simulink model "x20240109_HVDCMMCInterconnection"  (R2023b)
settings: Solver=FixedStepDiscrete  StartTime=0.0  StopTime=2  FixedStep=Ts_Power  RelTol=1e-4  EnableMultiTasking=on
PreLoadFcn:
  | HVDCMMCInterconnectionParam
StartFcn:
  | tic
StopFcn:
  | toc
values from neighbouring files (symbols this model uses):
  C_PM = 1.758e-3    (= 0.001758)    [HVDCMMCInterconnectionParam.m]
  Cg = 50e-9    (= 5e-08)    [HVDCMMCInterconnectionParam.m]
  D_R = 0.001    [HVDCMMCInterconnectionParam.m]
  D_Rs = 1e8    (= 100000000)    [HVDCMMCInterconnectionParam.m]
  D_Vf = 0    [HVDCMMCInterconnectionParam.m]
  Fnom = 50    [HVDCMMCInterconnectionParam.m]
  HRM = 2    [HVDCMMCInterconnectionParam.m]
  Ki_Ireg = 6    [HVDCMMCInterconnectionParam.m]
  Ki_Preg = 1.0    (= 1)    [HVDCMMCInterconnectionParam.m]
  Ki_Qreg = 1.0    (= 1)    [HVDCMMCInterconnectionParam.m]
  Ki_VDCreg = 100    [HVDCMMCInterconnectionParam.m]
  Kp_Ireg = 0.6    [HVDCMMCInterconnectionParam.m]
  Kp_Preg = 0.5/3    (= 0.166666666667)    [HVDCMMCInterconnectionParam.m]
  Kp_Qreg = 0.5/3    (= 0.166666666667)    [HVDCMMCInterconnectionParam.m]
  Kp_VDCreg = 4    [HVDCMMCInterconnectionParam.m]
  L_cable = 15e-3    (= 0.015)    [HVDCMMCInterconnectionParam.m]
  Larm = Larm_pu*(Zb_ac/(2*pi*Fnom))    [HVDCMMCInterconnectionParam.m]
  Lff = Larm_pu/2    (= 0.075)    [HVDCMMCInterconnectionParam.m]
  Limits_Ireg = [ 2.0  -2.0]    [HVDCMMCInterconnectionParam.m]
  Limits_Preg = [ 1.2, 0.8 ]    [HVDCMMCInterconnectionParam.m]
  Limits_Qreg = [ 0.25, -0.25 ]    [HVDCMMCInterconnectionParam.m]
  Limits_VDCreg = [ 2.0  -2.0]    [HVDCMMCInterconnectionParam.m]
  Lxfo = 0.12    [HVDCMMCInterconnectionParam.m]
  Nb_PM = 36    [HVDCMMCInterconnectionParam.m]
  Pnom = 1000e6    (= 1000000000)    [HVDCMMCInterconnectionParam.m]
  R_cable = 0.5    [HVDCMMCInterconnectionParam.m]
  R_startup = 400    [HVDCMMCInterconnectionParam.m]
  Rarm = Rarm_pu*Zb_ac    [HVDCMMCInterconnectionParam.m]
  Rff = Rarm_pu/2    (= 0.00075)    [HVDCMMCInterconnectionParam.m]
  Rg = 100    [HVDCMMCInterconnectionParam.m]
  Rxfo = 0.003    [HVDCMMCInterconnectionParam.m]
  Slope_Pref = 0.5    [HVDCMMCInterconnectionParam.m]
  Slope_Qref = 0.5    [HVDCMMCInterconnectionParam.m]
  Slope_Vdc_ref = Vnom_dc/5    (= 128000)    [HVDCMMCInterconnectionParam.m]
  Tbrk1_On = 0.1    [HVDCMMCInterconnectionParam.m]
  Tbrk2_On = 1.0    (= 1)    [HVDCMMCInterconnectionParam.m]
  Tdeblock = 1.5    [HVDCMMCInterconnectionParam.m]
  Tfault = 9999    [HVDCMMCInterconnectionParam.m]
  Ton_Converter2 = 4    [HVDCMMCInterconnectionParam.m]
  Ton_PQreg = 4    [HVDCMMCInterconnectionParam.m]
  Ton_VDCreg = 1.5    [HVDCMMCInterconnectionParam.m]
  Ts = Ts_Control    (= 4e-05)    [HVDCMMCInterconnectionParam.m]
  Ts_Control = 40e-6    (= 4e-05)    [HVDCMMCInterconnectionParam.m]
  Ts_Power = 20e-6    (= 2e-05)    [HVDCMMCInterconnectionParam.m]
  Vb_ac = sqrt(2/3)*Vnom_sec    [HVDCMMCInterconnectionParam.m]
  Vb_dc = Vnom_dc    (= 640000)    [HVDCMMCInterconnectionParam.m]
  Vc0_PM = 0    [HVDCMMCInterconnectionParam.m]
  Vnom_dc = 640e3    (= 640000)    [HVDCMMCInterconnectionParam.m]
  Vnom_prim = 400e3    (= 400000)    [HVDCMMCInterconnectionParam.m]
  Vnom_sec = 333e3    (= 333000)    [HVDCMMCInterconnectionParam.m]
  w = 2*pi*Fnom    (= 314.159265359)    [HVDCMMCInterconnectionParam.m]
undefined symbols (not defined in the file or in its folder): DiscIntNeverNeededParam, gcbh, Pcc, S, sps_AC, sps_ACDC2, sps_rtmsupport
libraries: simulink x48, spsControlledVoltageSourceLib x30, spsCurrentMeasurementLib x30, MMC_Lib x30, spsDiodeLib x20, spsSeriesRLCBranchLib x14, powerlib_extras x12, spsVoltageMeasurementLib x12, spsSecondOrderFilterLib x8, spsabctodq0Lib x8, spsGroundLib x7, spsMeanLib x4
(part 7 of 9)

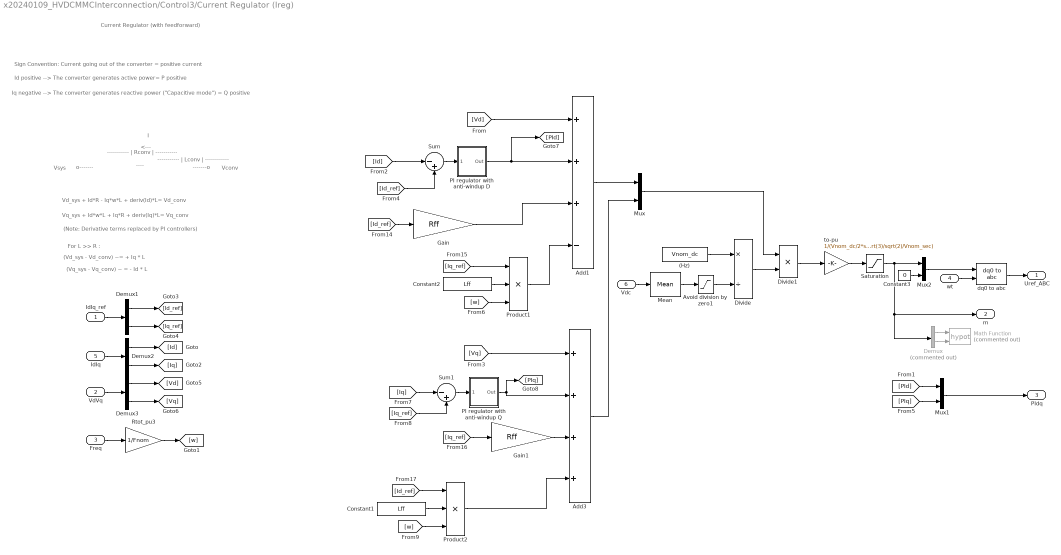
== system x20240109_HVDCMMCInterconnection/Control3/Current Regulator (Ireg) ==
  note: -----------
      | | Lconv |
      | ------------
  note: <---
  note: -------o
  note: Vconv
  note: ----
  note: -----------
      | | Rconv |
      | -----------
  note: For L >> R :
  note: (Vq_sys - Vq_conv) ~ = - Id * L
  note: (Vd_sys - Vd_conv) ~= + Iq * L
  note: Id positive --> The converter generates active power= P positive
  note: Iq negative --> The converter generates reactive power ("Capacitive mode") = Q positive
  note: Sign Convention: Current going out of the converter = positive current
  note: Current Regulator
      | (with feedforward)
  note: Vq_sys + Id*w*L + Iq*R + deriv(Iq)*L= Vq_conv
  note: Vd_sys + Id*R - Iq*w*L + deriv(Id)*L= Vd_conv
  note: (Note: Derivative terms replaced by PI controllers)
  note: Vsys
  note: o-------
  note: I
  IdIq_ref : Inport  PortDimensions=2
  VdVq : Inport  Port=2  PortDimensions=2
  Freq : Inport  Port=3  PortDimensions=1
  wt : Inport  Port=4  PortDimensions=1
  IdIq : Inport  Port=5  PortDimensions=2
  Vdc : Inport  Port=6  PortDimensions=1
  " (Hz)" : Constant  Value=Vnom_dc  SampleTime=Ts
  Add1 : Sum  Inputs=+++-
  Add3 : Sum  Inputs=++++
  Avoid division by zero1 : Saturate  UpperLimit=Vnom_dc*1.25  LowerLimit=Vnom_dc*0.75
  Constant1 : Constant  Value=Lff  SampleTime=Ts_Control
  Constant2 : Constant  Value=Lff  SampleTime=Ts_Control
  Constant3 : Constant  Value=0  SampleTime=Ts
  Demux : Demux  Commented=on  Outputs=2
  Demux1 : Demux  Outputs=2
  Demux2 : Demux  Outputs=2
  Demux3 : Demux  Outputs=2
  Divide : Product  Inputs=*/
  Divide1 : Product  Inputs=**
  Gain : Gain  Gain=Rff
  Gain1 : Gain  Gain=Rff
  Math Function : Math  Commented=on  Operator=hypot  SignedPower=on
  Mean : spsMeanLib/Mean  Freq=Fnom/3  Vinit=Vnom_dc  Ts=Ts
  Mux : Mux  Inputs=2
  Mux1 : Mux  Inputs=2
  Mux2 : Mux  Inputs=[2 1]
  PI regulator with anti-windup D : Subsystem  DialogController=POWERSYS.PowerSysDialog  mask(Discrete PI Controller){Kp=Kp_Ireg, Ki=Ki_Ireg, Par_Limits=Limits_Ireg, Init=0, Ts=Ts}
      mask prompts: Kp "Proportional gain (Kp):"; Ki "Integral gain (Ki):"; Par_Limits "Output limits: [ Upper   Lower ]"; Init "Output initial value:"; Ts "Sample time:"
      mask help: This block implements a discrete PI controller.
      mask init:
      | UpperLimit=Par_Limits(1);
      | LowerLimit=Par_Limits(2);
      | power_initmask();
      mask Help: This block is part of a subset of blocks in the Extras library that does not have documentation associated with it, other than the block mask description.
      mask Display: disp('PI');
  PI regulator with anti-windup Q : Subsystem  DialogController=POWERSYS.PowerSysDialog  mask(Discrete PI Controller){Kp=Kp_Ireg, Ki=Ki_Ireg, Par_Limits=Limits_Ireg, Init=0, Ts=Ts}
      mask prompts: Kp "Proportional gain (Kp):"; Ki "Integral gain (Ki):"; Par_Limits "Output limits: [ Upper   Lower ]"; Init "Output initial value:"; Ts "Sample time:"
      mask help: This block implements a discrete PI controller.
      mask init:
      | UpperLimit=Par_Limits(1);
      | LowerLimit=Par_Limits(2);
      | power_initmask();
      mask Help: This block is part of a subset of blocks in the Extras library that does not have documentation associated with it, other than the block mask description.
      mask Display: disp('PI');
  Product1 : Product  Inputs=3  RndMeth=Zero
  Product2 : Product  Inputs=3  RndMeth=Zero
  Rtot_pu3 : Gain  Gain=1/Fnom  SaturateOnIntegerOverflow=on  OutDataTypeStr=Inherit: Same as input  ParamDataTypeStr=Inherit: Same as input
  Saturation : Saturate  UpperLimit=Limits_Ireg(1)  LowerLimit=Limits_Ireg(2)
  Sum : Sum  Inputs=|-+
  Sum1 : Sum  Inputs=|-+
  dq0 to abc : spsdq0toabcLib/dq0 to abc  Alignment=90 degrees behind phase A axis
  to-pu : Gain  Gain=1/(Vnom_dc/2*sqrt(3)/sqrt(2)/Vnom_sec)
  Uref_ABC : Outport
  m : Outport  Port=2
  PIdq : Outport  Port=3
  wires:
  wt/1 -> dq0 to abc/2
  to-pu/1 -> Saturation/1
  Mux/1 -> Divide1/1
  dq0 to abc/1 -> Uref_ABC/1
  Divide/1 -> Divide1/2
  Mean/1 -> Avoid division by zero1/1
  Divide1/1 -> to-pu/1
  " (Hz)"/1 -> Divide/1
  Vdc/1 -> Mean/1
  Avoid division by zero1/1 -> Divide/2
  Mux1/1 -> PIdq/1
  Constant3/1 -> Mux2/2
  Mux2/1 -> dq0 to abc/1
  Demux/2 -> Math Function/2
  Demux/1 -> Math Function/1
  Saturation/1 -> Mux2/1, m/1, Demux/1
  PI regulator with anti-windup D/1(Out) -> [PId], Add1/2
  PI regulator with anti-windup Q/1(Out) -> [PIq], Add3/2
  [Vd] -> Add1/1
  Product1/1 -> Add1/4
  Gain/1 -> Add1/3
  Gain1/1 -> Add3/3
  Product2/1 -> Add3/4
  [Vq] -> Add3/1
  Demux2/1 -> [Id]
  IdIq/1 -> Demux2/1
  [Id_ref] -> Product2/1
  [Iq_ref] -> Gain1/1
  [Iq_ref] -> Product1/1
  [Id_ref] -> Gain/1
  [Id] -> Sum/1
  [Iq] -> Sum1/1
  Demux2/2 -> [Iq]
  [PIq] -> Mux1/2
  [PId] -> Mux1/1
  [w] -> Product1/3
  Constant2/1 -> Product1/2
  [w] -> Product2/3
  Constant1/1 -> Product2/2
  [Iq_ref] -> Sum1/2
  Sum1/1 -> PI regulator with anti-windup Q/1(Error)
  [Id_ref] -> Sum/2
  Sum/1 -> PI regulator with anti-windup D/1(Error)
  VdVq/1 -> Demux3/1
  Demux3/2 -> [Vq]
  Demux3/1 -> [Vd]
  IdIq_ref/1 -> Demux1/1
  Demux1/2 -> [Iq_ref]
  Demux1/1 -> [Id_ref]
  Rtot_pu3/1 -> [w]
  Freq/1 -> Rtot_pu3/1
  Add1/1 -> Mux/1
  Add3/1 -> Mux/2

== system x20240109_HVDCMMCInterconnection/Control3/DC Voltage Regulator (VDCreg) ==
  note: VDC Regulator
  Vdc_ref : Inport  PortDimensions=1
  On : Inport  Port=2  PortDimensions=1
  Vdc_meas : Inport  Port=3  PortDimensions=1
  Discrete-Time Integrator : DiscreteIntegrator  SampleTime=Ts  LimitOutput=on  UpperSaturationLimit=Limits_VDCreg(1)  LowerSaturationLimit=Limits_VDCreg(2)  ICPrevOutput=DiscIntNeverNeededParam  ICPrevScaledInput=DiscIntNeverNeededParam
  Product : Product  RndMeth=Zero
  Product1 : Product  RndMeth=Zero
  Rtot_pu2 : Gain  Gain=1/Vnom_dc  SaturateOnIntegerOverflow=on  OutDataTypeStr=Inherit: Same as input  ParamDataTypeStr=Inherit: Same as input
  Saturation2 : Saturate  UpperLimit=Limits_VDCreg(1)  LowerLimit=Limits_VDCreg(2)  SampleTime=Ts
  Sum : Sum  Inputs=|+-
  Sum6 : Sum  InputSameDT=on  SaturateOnIntegerOverflow=on  SampleTime=Ts  OutDataTypeStr=Inherit: Same as first input
  Switch1 : Switch  Criteria=u2 ~= 0  Threshold=0.5  OutDataTypeStr=double  SaturateOnIntegerOverflow=off  InputSameDT=off
  VdcNom_SM : Constant  Value=Kp_VDCreg
  VdcNom_SM1 : Constant  Value=Ki_VDCreg
  Zero-Order Hold : ZeroOrderHold  SampleTime=Ts
  Id_ref : Outport
  wires:
  Rtot_pu2/1 -> Product/2, Product1/2
  Saturation2/1 -> Id_ref/1
  VdcNom_SM/1 -> Product1/1
  Product/1 -> Discrete-Time Integrator/1
  Product1/1 -> Zero-Order Hold/1
  VdcNom_SM1/1 -> Product/1
  Sum6/1 -> Saturation2/1
  Discrete-Time Integrator/1 -> Sum6/2
  Zero-Order Hold/1 -> Sum6/1
  Vdc_ref/1 -> Sum/2, Switch1/3
  Switch1/1 -> Sum/1
  On/1 -> Switch1/2
  Sum/1 -> Rtot_pu2/1
  Vdc_meas/1 -> Switch1/1

== system x20240109_HVDCMMCInterconnection/Control3/PLL, Measurements and Transformation ==
  note: P (pu) = Vd*Id + Vq*Iq
  note: Q (pu) = Vq*Id - Vd*Iq
  note: P positive = Converter generates active power (Inverter Mode)
  note: Q positive = Converter generates reactive power (Capacitive Mode)
  Vabc : Inport  PortDimensions=3
  Iabc : Inport  Port=2  PortDimensions=3
  Add : Sum  Inputs=1
  Demux : Demux  Outputs=2
  Discrete Mean value : powerlib_extras/Discrete Measurements/Discrete  Mean value  Freq=Fnom  Vinit=0  Ts=Ts
  Discrete Mean value1 : powerlib_extras/Discrete Measurements/Discrete  Mean value  Freq=Fnom  Vinit=0  Ts=Ts
  I->pu2 : Gain  Gain=sqrt(3)*Vnom_sec/sqrt(2)/Pnom  SaturateOnIntegerOverflow=on  OutDataTypeStr=Inherit: Same as input  ParamDataTypeStr=Inherit: Same as input
  PLL (3ph) : spsPLL3phLib/PLL (3ph)  Fmin=0.9*Fnom  Par_Init=[0, Fnom]  ParK=[180, 3200, 1]  TcD=1e-4  MaxRateChangeFreq=12  FilterCutOffFreq=25  Ts=Ts  AGC=on
  Product : Product  RndMeth=Zero
  Product1 : Product  RndMeth=Zero
  Second-Order Filter : spsSecondOrderFilterLib/Second-Order Filter  FilterType=Lowpass  Fo=Fn_filter  Zeta=Zeta_filter  Ts=Ts  Initialize=off  Vac_Init="[0,  0,  60]"  Vdc_Init=0  PlotResponse=off  FreqRange=[0, 500, 1]
  Second-Order Filter1 : spsSecondOrderFilterLib/Second-Order Filter  FilterType=Lowpass  Fo=Fn_filter  Zeta=Zeta_filter  Ts=Ts  Initialize=off  Vac_Init="[0,  0,  60]"  Vdc_Init=0  PlotResponse=off  FreqRange=[0, 500, 1]
  Selector3 : Selector  InputPortWidth=2  IndexOptions=Index vector (dialog)  Indices=[2 1]  OutputSizes=1
  Selector4 : Selector  InputPortWidth=3  IndexOptions=Index vector (dialog)  Indices=[1 2]  OutputSizes=1
  Selector5 : Selector  InputPortWidth=3  IndexOptions=Index vector (dialog)  Indices=[1 2]  OutputSizes=1
  Subtract : Sum  Inputs=+-
  V->pu1 : Gain  Gain=1/(Vnom_sec/sqrt(3)*sqrt(2))  SaturateOnIntegerOverflow=on  OutDataTypeStr=Inherit: Same as input  ParamDataTypeStr=Inherit: Same as input
  abc to dq0 : spsabctodq0Lib/abc to dq0  Alignment=90 degrees behind phase A axis
  abc to dq1 : spsabctodq0Lib/abc to dq0  Alignment=90 degrees behind phase A axis
  Freq : Outport
  wt : Outport  Port=2
  IdIq : Outport  Port=3
  P : Outport  Port=4
  Q : Outport  Port=5
  VdVq : Outport  Port=6
  wires:
  Selector3/1 -> Product1/1
  Discrete Mean value1/1 -> Q/1
  Discrete Mean value/1 -> P/1
  Second-Order Filter/1 -> VdVq/1, Product/1, Selector3/1
  Second-Order Filter1/1 -> IdIq/1, Product1/2, Product/2
  Product/1 -> Add/1
  Product1/1 -> Demux/1
  Demux/1 -> Subtract/1
  Demux/2 -> Subtract/2
  Add/1 -> Discrete Mean value/1
  Subtract/1 -> Discrete Mean value1/1
  abc to dq0/1 -> Selector4/1
  PLL (3ph)/1 -> Freq/1
  V->pu1/1 -> abc to dq0/1, PLL (3ph)/1
  Vabc/1 -> V->pu1/1
  PLL (3ph)/2 -> wt/1, abc to dq1/2, abc to dq0/2
  Iabc/1 -> I->pu2/1
  abc to dq1/1 -> Selector5/1
  I->pu2/1 -> abc to dq1/1
  Selector4/1 -> Second-Order Filter/1
  Selector5/1 -> Second-Order Filter1/1

== system x20240109_HVDCMMCInterconnection/Control3/Reactive Power Regulator ==
  note: Reactive Power Regulator
  note: If PLL sync on Vprim --> Vq=0 --> Id = P/Vd et Iq = -1.0 * Q/Vd
  note: Q (pu) = Vq*Id - Vd*Iq (valid only for balanced & harmonics-free values)
  note: P (pu) = Vd*Id + Vq*Iq (Zero-sequence is not taken into account)
  On : Inport  PortDimensions=1
  Qref : Inport  Port=2  PortDimensions=1
  Qmes : Inport  Port=3  PortDimensions=1
  VdVq_mes : Inport  Port=4  PortDimensions=2
  Add2 : Sum
  Discrete Mean value1 : powerlib_extras/Discrete Measurements/Discrete  Mean value  Freq=Fnom  Vinit=0  Ts=Ts
  Discrete-Time Integrator : DiscreteIntegrator  SampleTime=Ts  LimitOutput=on  UpperSaturationLimit=Limits_Qreg(1)  LowerSaturationLimit=Limits_Qreg(2)  ICPrevOutput=DiscIntNeverNeededParam  ICPrevScaledInput=DiscIntNeverNeededParam
  Divide : Product  Inputs=*/
  Product : Product  RndMeth=Zero
  Product1 : Product  RndMeth=Zero
  Rtot_pu1 : Gain  Gain=-1  SaturateOnIntegerOverflow=on  OutDataTypeStr=Inherit: Same as input  ParamDataTypeStr=Inherit: Same as input
  Rtot_pu2 : Gain  Gain=-1  SaturateOnIntegerOverflow=on  OutDataTypeStr=Inherit: Same as input  ParamDataTypeStr=Inherit: Same as input
  Saturation : Saturate  UpperLimit=Limits_Qreg(1)  LowerLimit=Limits_Qreg(2)
  Saturation1 : Saturate  UpperLimit=2  LowerLimit=1e-6
  Saturation2 : Saturate  UpperLimit=Limits_Qreg(1)  LowerLimit=Limits_Qreg(2)
  Selector : Selector  InputPortWidth=2  IndexOptions=Index vector (dialog)  Indices=[1]  OutputSizes=1
  Sum : Sum  Inputs=|-+
  Sum6 : Sum  InputSameDT=on  SaturateOnIntegerOverflow=on  SampleTime=Ts  OutDataTypeStr=Inherit: Same as first input
  Switch1 : Switch  Criteria=u2 ~= 0  Threshold=0.5  OutDataTypeStr=double  SaturateOnIntegerOverflow=off  InputSameDT=off
  VdcNom_SM : Constant  Value=Kp_Qreg
  VdcNom_SM1 : Constant  Value=Ki_Qreg
  Zero-Order Hold : ZeroOrderHold  SampleTime=Ts
  Iq_ref : Outport
  wires:
  Saturation2/1 -> Rtot_pu1/1
  Saturation/1 -> Iq_ref/1
  Rtot_pu2/1 -> Add2/2
  Rtot_pu1/1 -> Add2/1
  Sum6/1 -> Saturation2/1
  Switch1/1 -> Product1/2, Product/2
  Sum/1 -> Switch1/1
  On/1 -> Switch1/2
  Add2/1 -> Saturation/1
  Product/1 -> Discrete-Time Integrator/1
  Product1/1 -> Zero-Order Hold/1
  VdcNom_SM/1 -> Product1/1
  VdcNom_SM1/1 -> Product/1
  Discrete-Time Integrator/1 -> Sum6/2
  Zero-Order Hold/1 -> Sum6/1
  Discrete Mean value1/1 -> Saturation1/1
  Saturation1/1 -> Divide/2
  Divide/1 -> Rtot_pu2/1
  Selector/1 -> Discrete Mean value1/1
  VdVq_mes/1 -> Selector/1
  Qmes/1 -> Sum/1
  Qref/1 -> Divide/1, Switch1/3, Sum/2

== system x20240109_HVDCMMCInterconnection/Discrete State-Space1/Discretize BE or Tustin ==
  note: Implement discretized state-space model using Tustin or TBE method
      |
      | BE      -> SM.DSSmethod=1
      | Tustin  -> SM.DSSmethod=2
      |
      |
      | Tustin
      | ------
      | Ad = inv(I - Ts/2*A)*(I + Ts/2*A)
      | Bd = inv(I - Ts/2*A)*B
      | Cd = C*inv(I - Ts/2*A)*Ts
      | Dd = C*inv(I - Ts/2*A)*B*Ts/2  + D  =  Cd*B/2+D
      |
      | TBE
      | ---
      | Ad = inv(I - Ts*A)
      | Bd = inv(I - Ts*A)*B
      | Cd = C*inv(I - Ts*A)*Ts
      | Dd = C*inv(I - Ts*A)*B*Ts  + D  =  Cd*B
      |
      | I = eye(SM.nState,SM.nState)
  A : Inport
  B : Inport  Port=2
  C : Inport  Port=3
  D : Inport  Port=4
  Add : Sum
  I : Constant  Value=eye(size(sps_AC.A,1))
  Product{1..4} (4 alike) : Product  Multiplication=Matrix(*)  SaturateOnIntegerOverflow=on  OutDataTypeStr=Inherit: Same as first input
  Sum1 : Sum  Inputs=+-  SaturateOnIntegerOverflow=on
  Sum5 : Sum  SaturateOnIntegerOverflow=on
  "Tustin: 1/2 BE : 1.0" : Gain  Gain=1/2  SaturateOnIntegerOverflow=on  OutDataTypeStr=Inherit: Same as input  ParamDataTypeStr=Inherit: Same as input
  "Tustin: Ts/2 BE : Ts" : Gain  Gain=Ts/2  SaturateOnIntegerOverflow=on  OutDataTypeStr=Inherit: Same as input  ParamDataTypeStr=Inherit: Same as input
  inversion : Product  Inputs=/  Multiplication=Matrix(*)  RndMeth=Zero
  wbase3 : Gain  Gain=Ts  SaturateOnIntegerOverflow=on  OutDataTypeStr=Inherit: Same as input  ParamDataTypeStr=Inherit: Same as input
  Ad : Outport  VectorParamsAs1DForOutWhenUnconnected=off
  Bd : Outport  Port=2  VectorParamsAs1DForOutWhenUnconnected=off
  Cd : Outport  Port=3  VectorParamsAs1DForOutWhenUnconnected=off
  Dd : Outport  Port=4  VectorParamsAs1DForOutWhenUnconnected=off
  wires:
  wbase3/1 -> Product3/1, Cd/1  "Cd"
  Product2/1 -> wbase3/1
  "Tustin: 1/2 BE : 1.0"/1 -> Add/1
  Product3/1 -> "Tustin: 1/2 BE : 1.0"/1
  C/1 -> Product2/1
  B/1 -> Product3/2, Product1/2
  Product1/1 -> Bd/1
  Sum5/1 -> Product4/2  "(I+Ts/2*A)"
  inversion/1 -> Product4/1, Product1/1, Product2/2  "INV"
  Sum1/1 -> inversion/1
  I/1 -> Sum1/1, Sum5/1  "I"
  A/1 -> "Tustin: Ts/2 BE : Ts"/1
  Product4/1 -> Ad/1
  "Tustin: Ts/2 BE : Ts"/1 -> Sum5/2, Sum1/2
  Add/1 -> Dd/1
  D/1 -> Add/2

== system x20240109_HVDCMMCInterconnection/Discrete State-Space1/Ihistory_Flux ==
  u : Inport
  Ad : Inport  Port=2
  Bd : Inport  Port=3
  Cd : Inport  Port=4
  D : Inport  Port=5
  Add : Sum
  Add2 : Sum
  Delay : Delay  DelayLength=1  InitialCondition=InitVec  SampleTime=dt
  Gain1 : Gain  Gain=exp(comp)
  Gain2 : Gain  Gain=exp(comp)
  Product{1..2,5,7} (4 alike) : Product  Multiplication=Matrix(*)  SaturateOnIntegerOverflow=on  OutDataTypeStr=Inherit: Same as first input
  Ihyst : Outport  VectorParamsAs1DForOutWhenUnconnected=off
  wires:
  Gain2/1 -> Product7/2  "xd"
  Gain1/1 -> Product2/2, Product5/2  "xd"
  Add2/1 -> Ihyst/1
  Bd/1 -> Product1/1  "u"
  u/1 -> Gain2/1, Product1/2  "u"
  Product2/1 -> Add2/1
  Product1/1 -> Add/1  "Bd*U"
  Add/1 -> Delay/1
  Delay/1 -> Gain1/1  "xd"
  Product5/1 -> Add/2  "Ad*X"
  Ad/1 -> Product5/1
  Cd/1 -> Product2/1
  Product7/1 -> Add2/2  "xd"
  D/1 -> Product7/1  "xd"

== system x20240109_HVDCMMCInterconnection/MMC/An ==
  Uref : Inport
  Add1 : Sum  Commented=on  Inputs=+-
  Add2 : Sum  Commented=on  Inputs=-+
  An_Db : spsDiodeLib/Diode  Ron=D_R  Lon=0  Vf=D_Vf  IC=0  UseSnubber=0  Rs=D_Rs  Cs=D_Cs  Measurements=on
  An_Dt : spsDiodeLib/Diode  Ron=D_R  Lon=0  Vf=D_Vf  IC=0  UseSnubber=0  Rs=D_Rs  Cs=D_Cs  Measurements=on
  An_Icap : spsCurrentMeasurementLib/Current Measurement  PhasorSimulation=off  OutputType=Complex  PSBequivalent=0
  An_Ipos : spsCurrentMeasurementLib/Current Measurement  PhasorSimulation=off  OutputType=Complex  PSBequivalent=0
  An_Vbl : spsControlledVoltageSourceLib/Controlled Voltage Source  Initialize=on  Source_Type=AC  Amplitude=0  Phase=0  Frequency=0  Measurements=None
  An_Vin : spsControlledVoltageSourceLib/Controlled Voltage Source  Initialize=on  Source_Type=AC  Amplitude=0  Phase=0  Frequency=0  Measurements=None
  Bus Selector1 : BusSelector  OutputSignals=Diode current
  Bus Selector2 : BusSelector  OutputSignals=Diode current
  Compare To Constant1 : simulink/Logic and Bit Operations/Compare To Constant  Commented=on  relop=<=  const=0.5  OutDataTypeStr=boolean
  Constant3 : Constant  Commented=on  Value=ones(1,1)
  Constant4 : Constant  Commented=on  Value=ones(1,1)
  Data Type Conversion2 : DataTypeConversion  Commented=on  OutDataTypeStr=double  SaturateOnIntegerOverflow=off  RndMeth=Floor
  Demux : Demux  Outputs=2
  Demux2 : Demux  Outputs=2
  Demux5 : Demux  Outputs=2
  Discrete-Time Integrator1 : DiscreteIntegrator  IntegratorMethod=Integration: Trapezoidal  gainval=1  InitialCondition=Vc_Initial  SampleTime=Ts  UpperSaturationLimit=5000  LowerSaturationLimit=500  ICPrevOutput=DiscIntNeverNeededParam  ICPrevScaledInput=DiscIntNeverNeededParam
  From11 : From  Commented=on  GotoTag=uref
  From13 : From  Commented=on  GotoTag=Blk  TagVisibility=global
  Gain1 : Gain  Gain=n
  Gain4 : Gain  Gain=1/(C*n)
  Gain5 : Gain  Gain=2
  Mux1 : Mux  Inputs=2
  Mux2 : Mux  Inputs=2
  Mux3 : Mux  Commented=on  Inputs=2
  Mux7 : Mux  Inputs=2
  Product1 : Product  Commented=on
  Product3 : Product
  Product4 : Product
  Product5 : Product  Commented=on
  Product7 : Product
  Saturation : Saturate  Commented=on  UpperLimit=1  LowerLimit=-1
  Scope : Scope  Commented=on  NumInputPorts=2
  Sum3 : Sum  Inputs=1  InputSameDT=on  SaturateOnIntegerOverflow=on  OutDataTypeStr=Inherit: Same as first input
  Sum4 : Sum  Inputs=+-  InputSameDT=on  SaturateOnIntegerOverflow=on  OutDataTypeStr=Inherit: Same as first input
  Unit Delay5 : UnitDelay  InitialCondition=Vc_Initial  SampleTime=Ts  HasFrameUpgradeWarning=on
  Unit Delay6 : UnitDelay  InitialCondition=Vc_Initial  SampleTime=Ts  HasFrameUpgradeWarning=on
  Unit Delay7 : UnitDelay  SampleTime=Ts  HasFrameUpgradeWarning=on
  An_pos : PMIOPort  Side=Left
  An_neg : PMIOPort  Port=2  Side=Left
  Vc : Outport  VectorParamsAs1DForOutWhenUnconnected=off
  tag scope: An_Vbl_EMT=global, An_Vin_EMT=global, I_An_Db_EMT=global, I_An_Dt_EMT=global
  wires:
  Demux/1 -> [An_Vin_EMT]
  [An_Vin_EMT] -> An_Vin/1
  Product3/1 -> Sum3/1
  Demux/2 -> [An_Vbl_EMT]
  [Ipos] -> Mux1/1
  Unit Delay5/1 -> Sum4/2
  Gain5/1 -> Sum4/1
  Sum4/1 -> Product7/2, Product4/2, Vc/1  "Vc"
  Discrete-Time Integrator1/1 -> Unit Delay6/1
  Mux2/1 -> Demux/1
  [An_Vbl_EMT] -> An_Vbl/1
  [Icap] -> Mux1/2
  Gain4/1 -> Discrete-Time Integrator1/1
  Unit Delay6/1 -> Gain5/1, Unit Delay5/1
  Mux1/1 -> Unit Delay7/1
  Mux7/1 -> Gain1/1
  Demux2/1 -> Product4/1
  Demux2/2 -> Product7/1
  Product4/1 -> Mux2/1  "Vin"
  Product7/1 -> Mux2/2  "Vbl"
  Demux5/2 -> [ublk]
  [uref] -> Mux7/1
  [ublk] -> Mux7/2
  An_Ipos/1 -> [Ipos]
  An_Icap/1 -> [Icap]
  Unit Delay7/1 -> Product3/2
  Gain1/1 -> Demux2/1, Product3/1
  Demux5/1 -> [uref]
  Uref/1 -> Demux5/1
  Data Type Conversion2/1 -> Product5/1, Product1/1
  From13/1 -> Compare To Constant1/1
  Add2/1 -> Add1/2, Product5/2
  Constant4/1 -> Add1/1
  From11/1 -> Saturation/1
  Compare To Constant1/1 -> Data Type Conversion2/1
  Add1/1 -> Product1/2
  Product1/1 -> Mux3/1
  Constant3/1 -> Add2/2
  Saturation/1 -> Add2/1
  Sum3/1 -> Gain4/1
  Product5/1 -> Mux3/2
  Bus Selector2/1 -> [I_An_Dt_EMT]  "<Diode current>"
  An_Dt/1 -> Bus Selector2/1
  Bus Selector1/1 -> [I_An_Db_EMT]  "<Diode current>"
  An_Db/1 -> Bus Selector1/1
  connections:
  An_Ipos/RConn1 -- An_Dt/LConn1 -- An_Db/RConn1
  An_Vbl/LConn1 -- An_neg/RConn1 -- An_Db/LConn1
  An_Vbl/RConn1 -- An_Icap/RConn1
  An_Dt/RConn1 -- An_Icap/LConn1
  An_pos/RConn1 -- An_Vin/RConn1
  An_Vin/LConn1 -- An_Ipos/LConn1

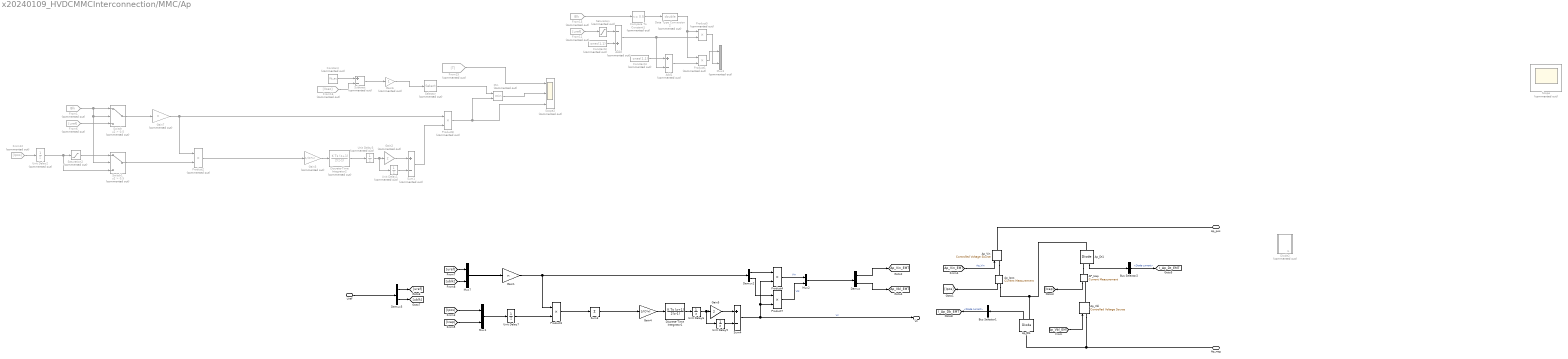
== system x20240109_HVDCMMCInterconnection/MMC/Ap ==
  Uref : Inport
  AP_Icap : spsCurrentMeasurementLib/Current Measurement  PhasorSimulation=off  OutputType=Complex  PSBequivalent=0
  Add1 : Sum  Commented=on  Inputs=+-
  Add2 : Sum  Commented=on  Inputs=-+
  Ap_Db : spsDiodeLib/Diode  Ron=D_R  Lon=0  Vf=D_Vf  IC=0  UseSnubber=0  Rs=D_Rs  Cs=D_Cs  Measurements=on
  Ap_Dt1 : spsDiodeLib/Diode  Ron=D_R  Lon=0  Vf=D_Vf  IC=0  UseSnubber=0  Rs=D_Rs  Cs=D_Cs  Measurements=on
  Ap_Ipos : spsCurrentMeasurementLib/Current Measurement  PhasorSimulation=off  OutputType=Complex  PSBequivalent=0
  Ap_Vbl : spsControlledVoltageSourceLib/Controlled Voltage Source  Initialize=on  Source_Type=AC  Amplitude=0  Phase=0  Frequency=0  Measurements=None
  Ap_Vin : spsControlledVoltageSourceLib/Controlled Voltage Source  Initialize=on  Source_Type=AC  Amplitude=0  Phase=0  Frequency=0  Measurements=None
  Bus Selector1 : BusSelector  OutputSignals=Diode current
  Bus Selector2 : BusSelector  OutputSignals=Diode current
  Compare To Constant1 : simulink/Logic and Bit Operations/Compare To Constant  Commented=on  relop=<=  const=0.5  OutDataTypeStr=boolean
  Constant : Constant  Commented=on  Value=Vb_ac
  Constant3 : Constant  Commented=on  Value=ones(1,1)
  Constant4 : Constant  Commented=on  Value=ones(1,1)
  Data Type Conversion2 : DataTypeConversion  Commented=on  OutDataTypeStr=double  SaturateOnIntegerOverflow=off  RndMeth=Floor
  Demux : Demux  Outputs=2
  Demux2 : Demux  Outputs=2
  Demux5 : Demux  Outputs=2
  Diode2 : Subsystem  Commented=on  AncestorBlock=sps_lib/Power Electronics/Diode2  DialogController=POWERSYS.PowerSysDialog  LoadFcn=sps_rtmsupport('LoadFcn',gcbh);  StartFcn=sps_rtmsupport('StartFcn',gcbh);  StopFcn=sps_rtmsupport('StopFcn',gcbh);  mask(Diode){Ron=D_R, Lon=0, Vf=D_Vf, IC=0, UseSnubber=0, Rs=D_Rs, Cs=inf, Measurements=on}
      mask prompts: Ron "Resistance Ron (Ohms) :"; Lon "Inductance Lon (H) :"; Vf "Forward voltage Vf (V) :"; IC "Initial current Ic (A) :"; UseSnubber "Snubber"; Rs "Snubber resistance Rs (Ohms) :"; Cs "Snubber capacitance Cs (F) :"; Measurements "Show measurement port"
      mask help:
      | Implements a diode in parallel with a series RC snubber circuit.
      | In on-state the Diode model has an internal resistance (Ron) and inductance (Lon).
      | For most applications the internal inductance should be set to zero.
      | The Diode impedance is infinite in off-state mode.
      mask init:
      | block = gcb;
      | [WantBlockChoice,Ts,X,Y,Ron,Vf] = powericon('SwitchesInit','Diode',block,Rs,Cs,Ron,Vf);
      | powericon('SetInternalModels','set',block,WantBlockChoice);
      settings: LibrarySourceBlock=sps_lib/Power Electronics/Diode2  CopyFcn=sps_rtmsupport('CopyFcn',gcbh); powericon('SwitchesCopyFcn','Diode',gcb)  DeleteFcn=sps_rtmsupport('DeleteFcn',gcbh);  UndoDeleteFcn=sps_rtmsupport('UndoDeleteFcn',gcbh);  ModelCloseFcn=sps_rtmsupport('ModelCloseFcn',gcbh);  PreSaveFcn=sps_rtmsupport('PreSaveFcn',gcbh);  PostSaveFcn=sps_rtmsupport('PostSaveFcn',gcbh);  NameChangeFcn=sps_rtmsupport('NameChangeFcn',gcbh);  PreCopyFcn=sps_rtmsupport('PreCopyFcn',gcbh);  OpenFcn=sps_rtmsupport('OpenFcn',gcbh, [5 8]);  CloseFcn=sps_rtmsupport('CloseFcn',gcbh);  PreDeleteFcn=sps_rtmsupport('PreDeleteFcn',gcbh);
      mask Help: helpview(psbhelp);
      mask Callback Ron: powericon('SwitchesEnables',gcb,'Diode');
      mask Callback Measurements:
      | powericon('OutputMCback',gcb);
      | %sps_rtmsupport('parametereditingmodes',gcbh, [5 8]);
      mask Display: plot(X.p1,Y.p1,X.p2,Y.p2,X.p3,Y.p3,X.p4,Y.p4,X.p5,Y.p5,X.p6,Y.p6)
  Discrete-Time Integrator1 : DiscreteIntegrator  IntegratorMethod=Integration: Trapezoidal  gainval=1  InitialCondition=Vc_Initial  SampleTime=Ts  UpperSaturationLimit=5000  LowerSaturationLimit=500  ICPrevOutput=DiscIntNeverNeededParam  ICPrevScaledInput=DiscIntNeverNeededParam
  Discrete-Time Integrator2 : DiscreteIntegrator  Commented=on  IntegratorMethod=Integration: Trapezoidal  gainval=1  InitialCondition=Vc_Initial  SampleTime=Ts  UpperSaturationLimit=5000  LowerSaturationLimit=500  ICPrevOutput=DiscIntNeverNeededParam  ICPrevScaledInput=DiscIntNeverNeededParam
  From1 : From  Commented=on  GotoTag=Blk  TagVisibility=global
  From11 : From  Commented=on  GotoTag=uref
  From12 : From  Commented=on  GotoTag=Ipos
  From13 : From  Commented=on  GotoTag=Blk  TagVisibility=global
  From15 : From  Commented=on  GotoTag=T
  From16 : From  Commented=on  GotoTag=Vsec  TagVisibility=global
  From6 : From  Commented=on  GotoTag=uref
  Gain1 : Gain  Gain=n
  Gain2 : Gain  Commented=on  Gain=2
  Gain3 : Gain  Commented=on  Gain=1/(C*n)
  Gain4 : Gain  Gain=1/(C*n)
  Gain5 : Gain  Gain=2
  Gain6 : Gain  Commented=on
  Gain7 : Gain  Commented=on  Gain=n
  Min : MinMax  Commented=on  Inputs=2
  Mux1 : Mux  Inputs=2
  Mux2 : Mux  Inputs=2
  Mux3 : Mux  Commented=on  Inputs=2
  Mux7 : Mux  Inputs=2
  Product{1..2,5,8} (4 alike) : Product  Commented=on
  Product3 : Product
  Product4 : Product
  Product7 : Product
  Saturation : Saturate  Commented=on  UpperLimit=1  LowerLimit=-1
  Saturation2 : Saturate  Commented=on  UpperLimit=inf  LowerLimit=0
  Scope : Scope  Commented=on  NumInputPorts=2
  Scope2 : Scope  Commented=on  NumInputPorts=3
  Selector : Selector  Commented=on  InputPortWidth=3  IndexOptions=Index vector (dialog)  Indices=[1]  OutputSizes=1
  Subtract : Sum  Commented=on  Inputs=+-
  Sum1 : Sum  Commented=on  Inputs=+-  InputSameDT=on  SaturateOnIntegerOverflow=on  OutDataTypeStr=Inherit: Same as first input
  Sum3 : Sum  Inputs=1  InputSameDT=on  SaturateOnIntegerOverflow=on  OutDataTypeStr=Inherit: Same as first input
  Sum4 : Sum  Inputs=+-  InputSameDT=on  SaturateOnIntegerOverflow=on  OutDataTypeStr=Inherit: Same as first input
  Switch : Switch  Commented=on  Criteria=u2 > Threshold  Threshold=0.5  SaturateOnIntegerOverflow=off  InputSameDT=off
  Switch1 : Switch  Commented=on  Criteria=u2 > Threshold  Threshold=0.5  SaturateOnIntegerOverflow=off  InputSameDT=off
  Unit Delay1 : UnitDelay  Commented=on  InitialCondition=Vc_Initial  SampleTime=Ts  HasFrameUpgradeWarning=on
  Unit Delay2 : UnitDelay  Commented=on  SampleTime=Ts  HasFrameUpgradeWarning=on
  Unit Delay3 : UnitDelay  Commented=on  InitialCondition=Vc_Initial  SampleTime=Ts  HasFrameUpgradeWarning=on
  Unit Delay5 : UnitDelay  InitialCondition=Vc_Initial  SampleTime=Ts  HasFrameUpgradeWarning=on
  Unit Delay6 : UnitDelay  InitialCondition=Vc_Initial  SampleTime=Ts  HasFrameUpgradeWarning=on
  Unit Delay7 : UnitDelay  SampleTime=Ts  HasFrameUpgradeWarning=on
  Ap_pos : PMIOPort  Side=Left
  Ap_neg : PMIOPort  Port=2  Side=Left
  Vc : Outport  VectorParamsAs1DForOutWhenUnconnected=off
  tag scope: Ap_Vbl_EMT=global, Ap_Vin_EMT=global, I_Ap_Db_EMT=global, I_Ap_Dt_EMT=global
  wires:
  Demux/1 -> [Ap_Vin_EMT]
  [Ap_Vin_EMT] -> Ap_Vin/1  "Ap_Vin"
  Product3/1 -> Sum3/1
  Demux/2 -> [Ap_Vbl_EMT]
  [Ipos] -> Mux1/1
  Unit Delay5/1 -> Sum4/2
  Gain5/1 -> Sum4/1
  Sum4/1 -> Product7/2, Product4/2, Vc/1  "Vc"
  Discrete-Time Integrator1/1 -> Unit Delay6/1
  Mux2/1 -> Demux/1
  [Ap_Vbl_EMT] -> Ap_Vbl/1
  [Icap] -> Mux1/2
  Gain4/1 -> Discrete-Time Integrator1/1
  Unit Delay6/1 -> Gain5/1, Unit Delay5/1
  Mux1/1 -> Unit Delay7/1
  Mux7/1 -> Gain1/1
  Demux2/1 -> Product4/1
  Demux2/2 -> Product7/1
  Product4/1 -> Mux2/1  "Vin"
  Product7/1 -> Mux2/2  "Vbl"
  Demux5/2 -> [ublk]
  [uref] -> Mux7/1
  [ublk] -> Mux7/2
  Ap_Ipos/1 -> [Ipos]
  AP_Icap/1 -> [Icap]
  Unit Delay7/1 -> Product3/2
  Gain1/1 -> Demux2/1, Product3/1
  Demux5/1 -> [uref]
  Uref/1 -> Demux5/1
  Data Type Conversion2/1 -> Product5/1, Product1/1
  From13/1 -> Compare To Constant1/1
  Add2/1 -> Add1/2, Product5/2
  Constant4/1 -> Add1/1
  From11/1 -> Saturation/1
  Compare To Constant1/1 -> Data Type Conversion2/1
  Add1/1 -> Product1/2
  Product1/1 -> Mux3/1
  Constant3/1 -> Add2/2
  Saturation/1 -> Add2/1
  Sum3/1 -> Gain4/1
  Product5/1 -> Mux3/2
  From1/1 -> Switch1/2, Switch/2, Switch/1
  Saturation2/1 -> Switch1/1
  Gain7/1 -> Product2/1, Product8/1
  Unit Delay3/1 -> Gain2/1, Unit Delay1/1
  Sum1/1 -> Product8/2
  Switch/1 -> Gain7/1
  Switch1/1 -> Product2/2
  From6/1 -> Switch/3
  Unit Delay2/1 -> Saturation2/1, Switch1/3
  Gain3/1 -> Discrete-Time Integrator2/1
  Discrete-Time Integrator2/1 -> Unit Delay3/1
  Unit Delay1/1 -> Sum1/2
  From12/1 -> Unit Delay2/1
  Product2/1 -> Gain3/1
  Gain2/1 -> Sum1/1
  Product8/1 -> Min/2, Scope2/3
  From16/1 -> Subtract/2
  Constant/1 -> Subtract/1
  Subtract/1 -> Gain6/1
  Gain6/1 -> Selector/1
  Selector/1 -> Min/1
  Min/1 -> Scope2/2
  From15/1 -> Scope2/1
  Bus Selector1/1 -> [I_Ap_Db_EMT]  "<Diode current>"
  Ap_Db/1 -> Bus Selector1/1
  Ap_Dt1/1 -> Bus Selector2/1
  Bus Selector2/1 -> [I_Ap_Dt_EMT]  "<Diode current>"
  connections:
  Ap_Ipos/RConn1 -- Ap_Dt1/LConn1 -- Ap_Db/RConn1
  Ap_Vbl/LConn1 -- Ap_neg/RConn1 -- Ap_Db/LConn1
  Ap_Vbl/RConn1 -- AP_Icap/RConn1
  Ap_Dt1/RConn1 -- AP_Icap/LConn1
  Ap_pos/RConn1 -- Ap_Vin/RConn1
  Ap_Vin/LConn1 -- Ap_Ipos/LConn1

== system x20240109_HVDCMMCInterconnection/MMC/Bn ==
  Uref : Inport
  Bn_Db : spsDiodeLib/Diode  Ron=D_R  Lon=0  Vf=D_Vf  IC=0  UseSnubber=0  Rs=D_Rs  Cs=D_Cs  Measurements=on
  Bn_Dt : spsDiodeLib/Diode  Ron=D_R  Lon=0  Vf=D_Vf  IC=0  UseSnubber=0  Rs=D_Rs  Cs=D_Cs  Measurements=on
  Bn_Icap : spsCurrentMeasurementLib/Current Measurement  PhasorSimulation=off  OutputType=Complex  PSBequivalent=0
  Bn_Ipos : spsCurrentMeasurementLib/Current Measurement  PhasorSimulation=off  OutputType=Complex  PSBequivalent=0
  Bn_Vbl : spsControlledVoltageSourceLib/Controlled Voltage Source  Initialize=on  Source_Type=AC  Amplitude=0  Phase=0  Frequency=0  Measurements=None
  Bn_Vin : spsControlledVoltageSourceLib/Controlled Voltage Source  Initialize=on  Source_Type=AC  Amplitude=0  Phase=0  Frequency=0  Measurements=None
  Bus Selector1 : BusSelector  OutputSignals=Diode current
  Bus Selector2 : BusSelector  OutputSignals=Diode current
  Demux : Demux  Outputs=2
  Demux2 : Demux  Outputs=2
  Demux5 : Demux  Outputs=2
  Discrete-Time Integrator1 : DiscreteIntegrator  IntegratorMethod=Integration: Trapezoidal  gainval=1  InitialCondition=Vc_Initial  SampleTime=Ts  UpperSaturationLimit=5000  LowerSaturationLimit=500  ICPrevOutput=DiscIntNeverNeededParam  ICPrevScaledInput=DiscIntNeverNeededParam
  Gain1 : Gain  Gain=n
  Gain4 : Gain  Gain=1/(C*n)
  Gain5 : Gain  Gain=2
  Mux1 : Mux  Inputs=2
  Mux2 : Mux  Inputs=2
  Mux7 : Mux  Inputs=2
  Product3 : Product
  Product4 : Product
  Product7 : Product
  Sum3 : Sum  Inputs=1  InputSameDT=on  SaturateOnIntegerOverflow=on  OutDataTypeStr=Inherit: Same as first input
  Sum4 : Sum  Inputs=+-  InputSameDT=on  SaturateOnIntegerOverflow=on  OutDataTypeStr=Inherit: Same as first input
  Unit Delay5 : UnitDelay  InitialCondition=Vc_Initial  SampleTime=Ts  HasFrameUpgradeWarning=on
  Unit Delay6 : UnitDelay  InitialCondition=Vc_Initial  SampleTime=Ts  HasFrameUpgradeWarning=on
  Unit Delay7 : UnitDelay  SampleTime=Ts  HasFrameUpgradeWarning=on
  Bn_pos : PMIOPort  Side=Left
  Bn_neg : PMIOPort  Port=2  Side=Left
  Vc : Outport  VectorParamsAs1DForOutWhenUnconnected=off
  tag scope: Bn_Vbl_EMT=global, Bn_Vin_EMT=global, I_Bn_Db_EMT=global, I_Bn_Dt_EMT=global
  wires:
  Demux/1 -> [Bn_Vin_EMT]
  [Bn_Vin_EMT] -> Bn_Vin/1
  Product3/1 -> Sum3/1
  Demux/2 -> [Bn_Vbl_EMT]
  [Ipos] -> Mux1/1
  Unit Delay5/1 -> Sum4/2
  Gain5/1 -> Sum4/1
  Sum4/1 -> Product7/2, Product4/2, Vc/1  "Vc"
  Discrete-Time Integrator1/1 -> Unit Delay6/1
  Mux2/1 -> Demux/1
  [Bn_Vbl_EMT] -> Bn_Vbl/1
  [Icap] -> Mux1/2
  Gain4/1 -> Discrete-Time Integrator1/1
  Unit Delay6/1 -> Gain5/1, Unit Delay5/1
  Mux1/1 -> Unit Delay7/1
  Mux7/1 -> Gain1/1
  Demux2/1 -> Product4/1
  Demux2/2 -> Product7/1
  Product4/1 -> Mux2/1  "Vin"
  Product7/1 -> Mux2/2  "Vbl"
  Demux5/2 -> [ublk]
  [uref] -> Mux7/1
  [ublk] -> Mux7/2
  Bn_Ipos/1 -> [Ipos]
  Bn_Icap/1 -> [Icap]
  Unit Delay7/1 -> Product3/2
  Gain1/1 -> Demux2/1, Product3/1
  Demux5/1 -> [uref]
  Uref/1 -> Demux5/1
  Sum3/1 -> Gain4/1
  Bus Selector2/1 -> [I_Bn_Dt_EMT]  "<Diode current>"
  Bn_Dt/1 -> Bus Selector2/1
  Bus Selector1/1 -> [I_Bn_Db_EMT]  "<Diode current>"
  Bn_Db/1 -> Bus Selector1/1
  connections:
  Bn_Ipos/RConn1 -- Bn_Dt/LConn1 -- Bn_Db/RConn1
  Bn_Vbl/LConn1 -- Bn_neg/RConn1 -- Bn_Db/LConn1
  Bn_Vbl/RConn1 -- Bn_Icap/RConn1
  Bn_Dt/RConn1 -- Bn_Icap/LConn1
  Bn_pos/RConn1 -- Bn_Vin/RConn1
  Bn_Vin/LConn1 -- Bn_Ipos/LConn1

== system x20240109_HVDCMMCInterconnection/MMC/Bp ==
  Uref : Inport
  BP_Icap : spsCurrentMeasurementLib/Current Measurement  PhasorSimulation=off  OutputType=Complex  PSBequivalent=0
  Bp_Db : spsDiodeLib/Diode  Ron=D_R  Lon=0  Vf=D_Vf  IC=0  UseSnubber=0  Rs=D_Rs  Cs=D_Cs  Measurements=on
  Bp_Dt : spsDiodeLib/Diode  Ron=D_R  Lon=0  Vf=D_Vf  IC=0  UseSnubber=0  Rs=D_Rs  Cs=D_Cs  Measurements=on
  Bp_Ipos : spsCurrentMeasurementLib/Current Measurement  PhasorSimulation=off  OutputType=Complex  PSBequivalent=0
  Bp_Vbl : spsControlledVoltageSourceLib/Controlled Voltage Source  Initialize=on  Source_Type=AC  Amplitude=0  Phase=0  Frequency=0  Measurements=None
  Bp_Vin : spsControlledVoltageSourceLib/Controlled Voltage Source  Initialize=on  Source_Type=AC  Amplitude=0  Phase=0  Frequency=0  Measurements=None
  Bus Selector1 : BusSelector  OutputSignals=Diode current
  Bus Selector2 : BusSelector  OutputSignals=Diode current
  Demux : Demux  Outputs=2
  Demux2 : Demux  Outputs=2
  Demux5 : Demux  Outputs=2
  Discrete-Time Integrator1 : DiscreteIntegrator  IntegratorMethod=Integration: Trapezoidal  gainval=1  InitialCondition=Vc_Initial  SampleTime=Ts  UpperSaturationLimit=5000  LowerSaturationLimit=500  ICPrevOutput=DiscIntNeverNeededParam  ICPrevScaledInput=DiscIntNeverNeededParam
  Gain1 : Gain  Gain=n
  Gain4 : Gain  Gain=1/(C*n)
  Gain5 : Gain  Gain=2
  Mux1 : Mux  Inputs=2
  Mux2 : Mux  Inputs=2
  Mux7 : Mux  Inputs=2
  Product3 : Product
  Product4 : Product
  Product7 : Product
  Sum3 : Sum  Inputs=1  InputSameDT=on  SaturateOnIntegerOverflow=on  OutDataTypeStr=Inherit: Same as first input
  Sum4 : Sum  Inputs=+-  InputSameDT=on  SaturateOnIntegerOverflow=on  OutDataTypeStr=Inherit: Same as first input
  Unit Delay5 : UnitDelay  InitialCondition=Vc_Initial  SampleTime=Ts  HasFrameUpgradeWarning=on
  Unit Delay6 : UnitDelay  InitialCondition=Vc_Initial  SampleTime=Ts  HasFrameUpgradeWarning=on
  Unit Delay7 : UnitDelay  SampleTime=Ts  HasFrameUpgradeWarning=on
  Bp_pos : PMIOPort  Side=Left
  Bp_neg : PMIOPort  Port=2  Side=Left
  Vc : Outport  VectorParamsAs1DForOutWhenUnconnected=off
  tag scope: Bp_Vbl_EMT=global, Bp_Vin_EMT=global, I_Bp_Db_EMT=global, I_Bp_Dt_EMT=global
  wires:
  Demux/1 -> [Bp_Vin_EMT]
  [Bp_Vin_EMT] -> Bp_Vin/1
  Product3/1 -> Sum3/1
  Demux/2 -> [Bp_Vbl_EMT]
  [Ipos] -> Mux1/1
  Unit Delay5/1 -> Sum4/2
  Gain5/1 -> Sum4/1
  Sum4/1 -> Product7/2, Product4/2, Vc/1  "Vc"
  Discrete-Time Integrator1/1 -> Unit Delay6/1
  Mux2/1 -> Demux/1
  [Bp_Vbl_EMT] -> Bp_Vbl/1
  [Icap] -> Mux1/2
  Gain4/1 -> Discrete-Time Integrator1/1
  Unit Delay6/1 -> Gain5/1, Unit Delay5/1
  Mux1/1 -> Unit Delay7/1
  Mux7/1 -> Gain1/1
  Demux2/1 -> Product4/1
  Demux2/2 -> Product7/1
  Product4/1 -> Mux2/1  "Vin"
  Product7/1 -> Mux2/2  "Vbl"
  Demux5/2 -> [ublk]
  [uref] -> Mux7/1
  [ublk] -> Mux7/2
  Bp_Ipos/1 -> [Ipos]
  BP_Icap/1 -> [Icap]
  Unit Delay7/1 -> Product3/2
  Gain1/1 -> Demux2/1, Product3/1
  Demux5/1 -> [uref]
  Uref/1 -> Demux5/1
  Sum3/1 -> Gain4/1
  Bus Selector2/1 -> [I_Bp_Dt_EMT]  "<Diode current>"
  Bp_Db/1 -> Bus Selector1/1
  Bus Selector1/1 -> [I_Bp_Db_EMT]  "<Diode current>"
  Bp_Dt/1 -> Bus Selector2/1
  connections:
  Bp_Ipos/RConn1 -- Bp_Dt/LConn1 -- Bp_Db/RConn1
  Bp_Vbl/LConn1 -- Bp_neg/RConn1 -- Bp_Db/LConn1
  Bp_Vbl/RConn1 -- BP_Icap/RConn1
  Bp_Dt/RConn1 -- BP_Icap/LConn1
  Bp_pos/RConn1 -- Bp_Vin/RConn1
  Bp_Vin/LConn1 -- Bp_Ipos/LConn1

== system x20240109_HVDCMMCInterconnection/MMC/Cn ==
  Uref : Inport
  Bus Selector1 : BusSelector  OutputSignals=Diode current
  Bus Selector2 : BusSelector  OutputSignals=Diode current
  Cn_Db : spsDiodeLib/Diode  Ron=D_R  Lon=0  Vf=D_Vf  IC=0  UseSnubber=0  Rs=D_Rs  Cs=D_Cs  Measurements=on
  Cn_Dt : spsDiodeLib/Diode  Ron=D_R  Lon=0  Vf=D_Vf  IC=0  UseSnubber=0  Rs=D_Rs  Cs=D_Cs  Measurements=on
  Cn_Icap : spsCurrentMeasurementLib/Current Measurement  PhasorSimulation=off  OutputType=Complex  PSBequivalent=0
  Cn_Ipos : spsCurrentMeasurementLib/Current Measurement  PhasorSimulation=off  OutputType=Complex  PSBequivalent=0
  Cn_Vbl : spsControlledVoltageSourceLib/Controlled Voltage Source  Initialize=on  Source_Type=AC  Amplitude=0  Phase=0  Frequency=0  Measurements=None
  Cn_Vin : spsControlledVoltageSourceLib/Controlled Voltage Source  Initialize=on  Source_Type=AC  Amplitude=0  Phase=0  Frequency=0  Measurements=None
  Demux : Demux  Outputs=2
  Demux2 : Demux  Outputs=2
  Demux5 : Demux  Outputs=2
  Discrete-Time Integrator1 : DiscreteIntegrator  IntegratorMethod=Integration: Trapezoidal  gainval=1  InitialCondition=Vc_Initial  SampleTime=Ts  UpperSaturationLimit=5000  LowerSaturationLimit=500  ICPrevOutput=DiscIntNeverNeededParam  ICPrevScaledInput=DiscIntNeverNeededParam
  Gain1 : Gain  Gain=n
  Gain4 : Gain  Gain=1/(C*n)
  Gain5 : Gain  Gain=2
  Mux1 : Mux  Inputs=2
  Mux2 : Mux  Inputs=2
  Mux7 : Mux  Inputs=2
  Product3 : Product
  Product4 : Product
  Product7 : Product
  Sum3 : Sum  Inputs=1  InputSameDT=on  SaturateOnIntegerOverflow=on  OutDataTypeStr=Inherit: Same as first input
  Sum4 : Sum  Inputs=+-  InputSameDT=on  SaturateOnIntegerOverflow=on  OutDataTypeStr=Inherit: Same as first input
  Unit Delay5 : UnitDelay  InitialCondition=Vc_Initial  SampleTime=Ts  HasFrameUpgradeWarning=on
  Unit Delay6 : UnitDelay  InitialCondition=Vc_Initial  SampleTime=Ts  HasFrameUpgradeWarning=on
  Unit Delay7 : UnitDelay  SampleTime=Ts  HasFrameUpgradeWarning=on
  Cn_pos : PMIOPort  Side=Left
  Cn_neg : PMIOPort  Port=2  Side=Left
  Vc : Outport  VectorParamsAs1DForOutWhenUnconnected=off
  tag scope: Cn_Vbl_EMT=global, Cn_Vin_EMT=global, I_Cn_Db_EMT=global, I_Cn_Dt_EMT=global
  wires:
  Demux/1 -> [Cn_Vin_EMT]
  [Cn_Vin_EMT] -> Cn_Vin/1
  Product3/1 -> Sum3/1
  Demux/2 -> [Cn_Vbl_EMT]
  [Ipos] -> Mux1/1
  Unit Delay5/1 -> Sum4/2
  Gain5/1 -> Sum4/1
  Sum4/1 -> Product7/2, Product4/2, Vc/1  "Vc"
  Discrete-Time Integrator1/1 -> Unit Delay6/1
  Mux2/1 -> Demux/1
  [Cn_Vbl_EMT] -> Cn_Vbl/1
  [Icap] -> Mux1/2
  Gain4/1 -> Discrete-Time Integrator1/1
  Unit Delay6/1 -> Gain5/1, Unit Delay5/1
  Mux1/1 -> Unit Delay7/1
  Mux7/1 -> Gain1/1
  Demux2/1 -> Product4/1
  Demux2/2 -> Product7/1
  Product4/1 -> Mux2/1  "Vin"
  Product7/1 -> Mux2/2  "Vbl"
  Demux5/2 -> [ublk]
  [uref] -> Mux7/1
  [ublk] -> Mux7/2
  Cn_Ipos/1 -> [Ipos]
  Cn_Icap/1 -> [Icap]
  Unit Delay7/1 -> Product3/2
  Gain1/1 -> Demux2/1, Product3/1
  Demux5/1 -> [uref]
  Uref/1 -> Demux5/1
  Sum3/1 -> Gain4/1
  Bus Selector1/1 -> [I_Cn_Db_EMT]  "<Diode current>"
  Bus Selector2/1 -> [I_Cn_Dt_EMT]  "<Diode current>"
  Cn_Dt/1 -> Bus Selector2/1
  Cn_Db/1 -> Bus Selector1/1
  connections:
  Cn_Ipos/RConn1 -- Cn_Dt/LConn1 -- Cn_Db/RConn1
  Cn_Vbl/LConn1 -- Cn_neg/RConn1 -- Cn_Db/LConn1
  Cn_Vbl/RConn1 -- Cn_Icap/RConn1
  Cn_Dt/RConn1 -- Cn_Icap/LConn1
  Cn_pos/RConn1 -- Cn_Vin/RConn1
  Cn_Vin/LConn1 -- Cn_Ipos/LConn1

== system x20240109_HVDCMMCInterconnection/MMC/Cp ==
  Uref : Inport
  Bus Selector1 : BusSelector  OutputSignals=Diode current
  Bus Selector2 : BusSelector  OutputSignals=Diode current
  CP_Icap : spsCurrentMeasurementLib/Current Measurement  PhasorSimulation=off  OutputType=Complex  PSBequivalent=0
  Cp_Db : spsDiodeLib/Diode  Ron=D_R  Lon=0  Vf=D_Vf  IC=0  UseSnubber=0  Rs=D_Rs  Cs=D_Cs  Measurements=on
  Cp_Dt : spsDiodeLib/Diode  Ron=D_R  Lon=0  Vf=D_Vf  IC=0  UseSnubber=0  Rs=D_Rs  Cs=D_Cs  Measurements=on
  Cp_Ipos : spsCurrentMeasurementLib/Current Measurement  PhasorSimulation=off  OutputType=Complex  PSBequivalent=0
  Cp_Vbl : spsControlledVoltageSourceLib/Controlled Voltage Source  Initialize=on  Source_Type=AC  Amplitude=0  Phase=0  Frequency=0  Measurements=None
  Cp_Vin : spsControlledVoltageSourceLib/Controlled Voltage Source  Initialize=on  Source_Type=AC  Amplitude=0  Phase=0  Frequency=0  Measurements=None
  Demux : Demux  Outputs=2
  Demux2 : Demux  Outputs=2
  Demux5 : Demux  Outputs=2
  Discrete-Time Integrator1 : DiscreteIntegrator  IntegratorMethod=Integration: Trapezoidal  gainval=1  InitialCondition=Vc_Initial  SampleTime=Ts  UpperSaturationLimit=5000  LowerSaturationLimit=500  ICPrevOutput=DiscIntNeverNeededParam  ICPrevScaledInput=DiscIntNeverNeededParam
  Gain1 : Gain  Gain=n
  Gain4 : Gain  Gain=1/(C*n)
  Gain5 : Gain  Gain=2
  Mux1 : Mux  Inputs=2
  Mux2 : Mux  Inputs=2
  Mux7 : Mux  Inputs=2
  Product3 : Product
  Product4 : Product
  Product7 : Product
  Sum3 : Sum  Inputs=1  InputSameDT=on  SaturateOnIntegerOverflow=on  OutDataTypeStr=Inherit: Same as first input
  Sum4 : Sum  Inputs=+-  InputSameDT=on  SaturateOnIntegerOverflow=on  OutDataTypeStr=Inherit: Same as first input
  Unit Delay5 : UnitDelay  InitialCondition=Vc_Initial  SampleTime=Ts  HasFrameUpgradeWarning=on
  Unit Delay6 : UnitDelay  InitialCondition=Vc_Initial  SampleTime=Ts  HasFrameUpgradeWarning=on
  Unit Delay7 : UnitDelay  SampleTime=Ts  HasFrameUpgradeWarning=on
  Cp_pos : PMIOPort  Side=Left
  Cp_neg : PMIOPort  Port=2  Side=Left
  Vc : Outport  VectorParamsAs1DForOutWhenUnconnected=off
  tag scope: Cp_Vbl_EMT=global, Cp_Vin_EMT=global, I_Cp_Db_EMT=global, I_Cp_Dt_EMT=global
  wires:
  Demux/1 -> [Cp_Vin_EMT]
  [Cp_Vin_EMT] -> Cp_Vin/1
  Product3/1 -> Sum3/1
  Demux/2 -> [Cp_Vbl_EMT]
  [Ipos] -> Mux1/1
  Unit Delay5/1 -> Sum4/2
  Gain5/1 -> Sum4/1
  Sum4/1 -> Product7/2, Product4/2, Vc/1  "Vc"
  Discrete-Time Integrator1/1 -> Unit Delay6/1
  Mux2/1 -> Demux/1
  [Cp_Vbl_EMT] -> Cp_Vbl/1
  [Icap] -> Mux1/2
  Gain4/1 -> Discrete-Time Integrator1/1
  Unit Delay6/1 -> Gain5/1, Unit Delay5/1
  Mux1/1 -> Unit Delay7/1
  Mux7/1 -> Gain1/1
  Demux2/1 -> Product4/1
  Demux2/2 -> Product7/1
  Product4/1 -> Mux2/1  "Vin"
  Product7/1 -> Mux2/2  "Vbl"
  Demux5/2 -> [ublk]
  [uref] -> Mux7/1
  [ublk] -> Mux7/2
  Cp_Ipos/1 -> [Ipos]
  CP_Icap/1 -> [Icap]
  Unit Delay7/1 -> Product3/2
  Gain1/1 -> Demux2/1, Product3/1
  Demux5/1 -> [uref]
  Uref/1 -> Demux5/1
  Sum3/1 -> Gain4/1
  Bus Selector2/1 -> [I_Cp_Dt_EMT]  "<Diode current>"
  Cp_Db/1 -> Bus Selector1/1
  Bus Selector1/1 -> [I_Cp_Db_EMT]  "<Diode current>"
  Cp_Dt/1 -> Bus Selector2/1
  connections:
  Cp_Ipos/RConn1 -- Cp_Dt/LConn1 -- Cp_Db/RConn1
  Cp_Vbl/LConn1 -- Cp_neg/RConn1 -- Cp_Db/LConn1
  Cp_Vbl/RConn1 -- CP_Icap/RConn1
  Cp_Dt/RConn1 -- CP_Icap/LConn1
  Cp_pos/RConn1 -- Cp_Vin/RConn1
  Cp_Vin/LConn1 -- Cp_Ipos/LConn1

== system x20240109_HVDCMMCInterconnection/MMC/Half-Bridge MMC Ap (Aggregate model of 36 PM)2 ==
  Uref : Inport
  Controlled Voltage Source : spsControlledVoltageSourceLib/Controlled Voltage Source  Initialize=on  Source_Type=AC  Amplitude=0  Phase=0  Frequency=0  Measurements=None
  Controlled Voltage Source1 : spsControlledVoltageSourceLib/Controlled Voltage Source  Initialize=on  Source_Type=AC  Amplitude=0  Phase=0  Frequency=0  Measurements=None
  Current Measurement : spsCurrentMeasurementLib/Current Measurement  PhasorSimulation=off  OutputType=Complex  PSBequivalent=0
  Current Measurement1 : spsCurrentMeasurementLib/Current Measurement  PhasorSimulation=off  OutputType=Complex  PSBequivalent=0
  Demux : Demux  Outputs=2
  Diode : spsDiodeLib/Diode  Ron=Ron_Diode  Lon=0  Vf=Vf_Diode  IC=0  UseSnubber=0  Rs=Rs_Diode  Cs=Cs_Diode  Measurements=off
  Diode1 : spsDiodeLib/Diode  Ron=Ron_Diode  Lon=0  Vf=Vf_Diode  IC=0  UseSnubber=0  Rs=Rs_Diode  Cs=Cs_Diode  Measurements=off
  Discrete-Time Integrator1 : DiscreteIntegrator  IntegratorMethod=Integration: Trapezoidal  gainval=1  InitialCondition=Vc_Initial  SampleTime=Ts  UpperSaturationLimit=5000  LowerSaturationLimit=500  ICPrevOutput=DiscIntNeverNeededParam  ICPrevScaledInput=DiscIntNeverNeededParam
  Gain1 : Gain  Gain=n
  Gain4 : Gain  Gain=1/(C*n)
  Gain5 : Gain  Gain=2
  Mux1 : Mux  Inputs=2
  Product3 : Product
  Product4 : Product
  Sum3 : Sum  Inputs=1  InputSameDT=on  SaturateOnIntegerOverflow=on  OutDataTypeStr=Inherit: Same as first input
  Sum4 : Sum  Inputs=+-  InputSameDT=on  SaturateOnIntegerOverflow=on  OutDataTypeStr=Inherit: Same as first input
  Unit Delay2 : UnitDelay  SampleTime=Ts  HasFrameUpgradeWarning=on
  Unit Delay5 : UnitDelay  InitialCondition=Vc_Initial  SampleTime=Ts  HasFrameUpgradeWarning=on
  Unit Delay6 : UnitDelay  InitialCondition=Vc_Initial  SampleTime=Ts  HasFrameUpgradeWarning=on
  1 : PMIOPort  Side=Left
  2 : PMIOPort  Port=2  Side=Left
  Vc : Outport  VectorParamsAs1DForOutWhenUnconnected=off
  wires:
  Demux/1 -> [Vin]
  [Vin] -> Controlled Voltage Source/1
  Current Measurement1/1 -> [Icap]
  Product3/1 -> Sum3/1
  Demux/2 -> [Vbl]
  [Imod] -> Mux1/1
  Sum3/1 -> Gain4/1
  Unit Delay5/1 -> Sum4/2
  Gain5/1 -> Sum4/1
  Mux1/1 -> Unit Delay2/1
  Uref/1 -> Gain1/1
  Sum4/1 -> Vc/1, Product4/2
  Current Measurement/1 -> [Imod]
  Unit Delay2/1 -> Product3/2
  Discrete-Time Integrator1/1 -> Unit Delay6/1
  Product4/1 -> Demux/1
  [Vbl] -> Controlled Voltage Source1/1
  [Icap] -> Mux1/2
  Gain4/1 -> Discrete-Time Integrator1/1
  Unit Delay6/1 -> Gain5/1, Unit Delay5/1
  Gain1/1 -> Product3/1, Product4/1
  connections:
  Diode1/LConn1 -- Current Measurement/RConn1 -- Diode/RConn1
  Controlled Voltage Source1/LConn1 -- Diode/LConn1 -- 2/RConn1
  Controlled Voltage Source1/RConn1 -- Current Measurement1/RConn1
  Diode1/RConn1 -- Current Measurement1/LConn1
  1/RConn1 -- Controlled Voltage Source/RConn1
  Controlled Voltage Source/LConn1 -- Current Measurement/LConn1
